simulink subsystem "Szakasz"  (R2024b)
settings: Solver=VariableStepAuto  StartTime=0.0  StopTime=10.0  RelTol=1e-3
settings Model: Creator=Asus  LastModifiedBy=Asus

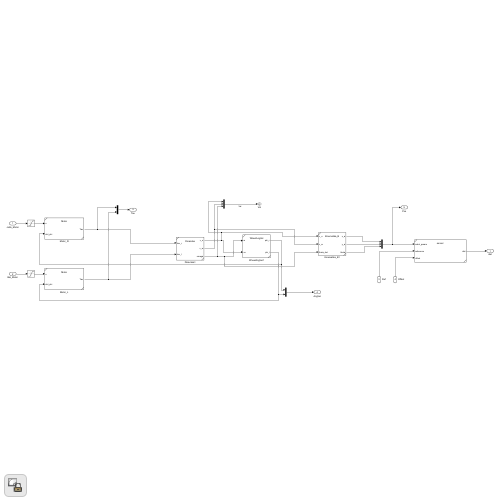
[thumbnail: Simulink's stored preview of the top-level diagram]
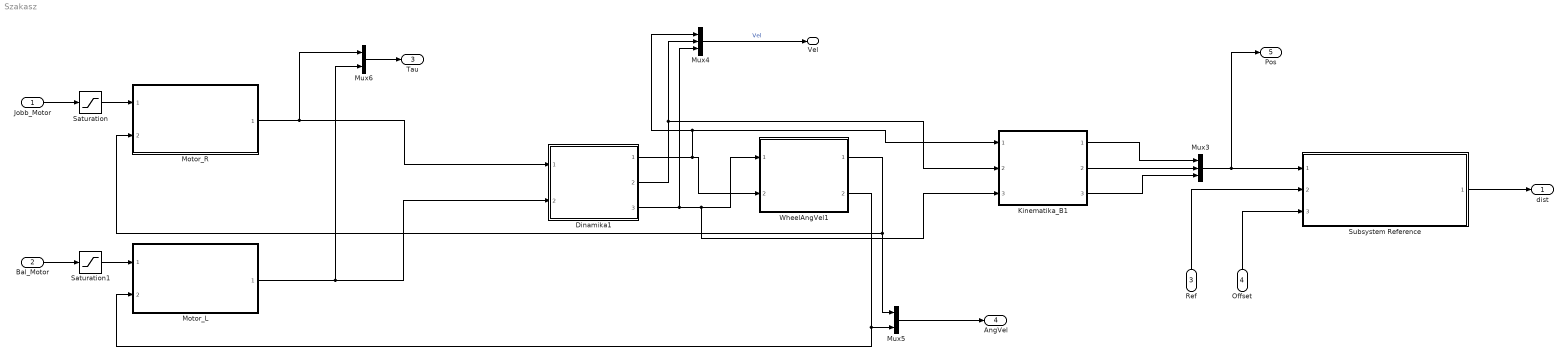
== system Szakasz ==
  Jobb_Motor : Inport
  Bal_Motor : Inport  Port=2
  Ref : Inport  Port=3
  Offset : Inport  Port=4
  Dinamika1 : Subsystem  ReferencedSubsystem=Dinamika
  Kinematika_B1 : Subsystem  ReferencedSubsystem=Kinematika_B
  Motor_L : Subsystem  ReferencedSubsystem=Motor
  Motor_R : Subsystem  ReferencedSubsystem=Motor
  Mux3 : Mux  Inputs=3
  Mux4 : Mux  Inputs=3
  Mux5 : Mux  Inputs=2
  Mux6 : Mux  Inputs=2
  Saturation : Saturate  UpperLimit=5  LowerLimit=-5
  Saturation1 : Saturate  UpperLimit=5  LowerLimit=-5
  Subsystem Reference : Subsystem  ReferencedSubsystem=sensor
  WheelAngVel1 : Subsystem  ReferencedSubsystem=WheelAngVel
  dist : Outport
  Vel : Outport  Port=2
  Tau : Outport  Port=3
  AngVel : Outport  Port=4
  Pos : Outport  Port=5
  wires:
  Jobb_Motor/1 -> Saturation/1
  Kinematika_B1/1 -> Mux3/1
  Dinamika1/2 -> Mux4/2, Kinematika_B1/2
  Mux6/1 -> Tau/1
  WheelAngVel1/2 -> Mux5/2, Motor_L/2
  Kinematika_B1/3 -> Mux3/3
  Dinamika1/3 -> WheelAngVel1/1, Kinematika_B1/3, Mux4/3
  Mux5/1 -> AngVel/1
  Motor_R/1 -> Dinamika1/1, Mux6/1
  Mux4/1 -> Vel/1  "Vel"
  Saturation/1 -> Motor_R/1
  WheelAngVel1/1 -> Motor_R/2, Mux5/1
  Motor_L/1 -> Dinamika1/2, Mux6/2
  Saturation1/1 -> Motor_L/1
  Dinamika1/1 -> WheelAngVel1/2, Kinematika_B1/1, Mux4/1
  Kinematika_B1/2 -> Mux3/2
  Bal_Motor/1 -> Saturation1/1
  Mux3/1 -> Pos/1, Subsystem Reference/1
  Ref/1 -> Subsystem Reference/2
  Offset/1 -> Subsystem Reference/3
  Subsystem Reference/1 -> dist/1
